simulink model "gm_PN_generator_Tx_mq"  (R2020a)
settings: Solver=FixedStepDiscrete  StartTime=0.0  StopTime=10  RelTol=1e-3
undefined symbols (not defined in the file): filt, Fs, ip, usb
libraries: commseqgen3 x2, dspmlti4 x2, plutoradiolib x1, commdigbbndpm3 x1, modelsimlib x1
settings Model: Creator=juanj  LastModifiedBy=juanj
settings OptimizationCC: BlockReduction=off  ConditionallyExecuteInputs=off  DefaultParameterBehavior=Inlined
settings DebuggingCC: AlgebraicLoopMsg=error  InheritedTsInSrcMsg=none  SingleTaskRateTransMsg=error  UnderSpecifiedDimensionMsg=warning
settings HardwareCC: ProdBitPerPointer=32  ProdBitPerSizeT=32  ProdBitPerPtrDiffT=32  ProdLargestAtomicFloat=None  ProdIntDivRoundTo=Undefined  ProdEndianess=Unspecified  ProdWordSize=32  ProdHWDeviceType=ASIC/FPGA->ASIC/FPGA  TargetBitPerPointer=64  TargetBitPerSizeT=64  TargetBitPerPtrDiffT=64  TargetLongLongMode=on  TargetIntDivRoundTo=Zero  TargetEndianess=LittleEndian  TargetWordSize=64  TargetHWDeviceType=Custom Processor->MATLAB Host Computer  ProdEqTarget=off

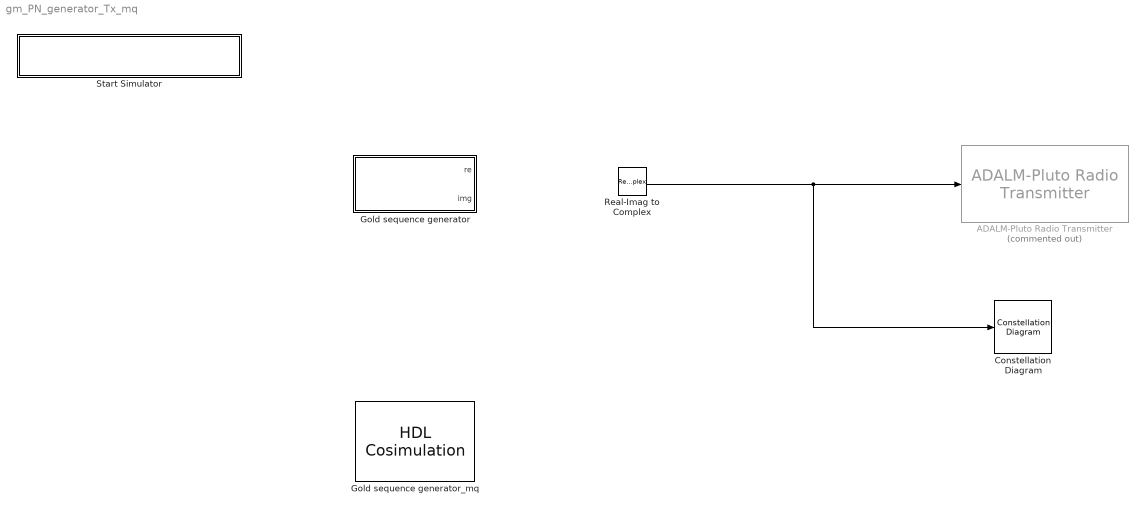
== system gm_PN_generator_Tx_mq ==
  ADALM-Pluto Radio Transmitter : plutoradiolib/ADALM-Pluto Radio Transmitter  Commented=on  RadioID=usb:0  uri=ip:10.0.0.200  CenterFrequencySource=Dialog  CenterFrequency=2.4e9  GainSource=Dialog  Gain=-10  ChannelMapping=1  BasebandSampleRate=1e6  UnderflowOutputPort=off  ShowAdvancedProperties=off  UseCustomFilter=off  filtPathRates=[737280000 11520000 3840000 1920000 960000 240000]  filtCoefficients=[-192 82 85 -215 228 -102 -110 290 -318 145 160 -426 471 -215 -238 633 -697 318 349 -923 1009 -457 -498 1309 -1423 640 693 -1812 1959 -876 -945 2458 -2647 1180 1268 -3290 3534 -1572 -1688 4375 -4698 2091 2247 -5836 6284 -2807 -3031 7918 -8588 3870 4225 -11182 12324 -5662 -6330 17255 -19735 9507 11312 -33568 43355 -25227 -42139 305542 305542 -42139 -25227 43355 -33568 11312 9507 -19735 17255 -6330 -5662 12324 -11182 4225 3870 -8588 7918 -3031 -2807 6284 -5836 2247 2091 -4698 4375 -1688 -1572 3534 -3290 1268 1180 -2647 2458 -945 -876 1959 -1812 693 640 -1423 1309 -498 -457 1009 -923 349 318 -697 633 -238 -215 471 -426 160 145 -318 290 -110 -102 228 -215 85 82 -192]  filtCoefficientSize=128  filtDecimInterpFactor=4  filtGain=-12  filtRFBandwidth=18000000  filterConfigStruct=struct()  DataSourceSelect=Input Port  DDSTone1Freq=5e3  DDSTone2Freq=10e3  DDSTone1Scale=0.5  DDSTone2Scale=0.25  DataTimeout=Inf  FrequencyCorrection=0  ENSMPinControlMode=None  BISTLoopbackMode=Disabled  BISTToneInject=Disabled  BISTSignalGen=PRBS  BISTToneFreq=Fs/32  BISTToneLevel=0
      settings: SourceProductBaseCode=PLUTO
  Constellation Diagram : ConstellationDiagram
  Gold sequence generator : Subsystem  TreatAsAtomicUnit=on
  Gold sequence generator_mq : modelsimlib/HDL Cosimulation  PortModes=[]  PortTimes=[]  PortSigns=[]  PortFracLengths=[]  CommLocal=on  CommSharedMemory=on  CommPortNumber=4449  CommShowInfo=on  ClockModes=[]  ClockTimes=[]  TclPreSimCommand=|  TclPostSimCommand="puts \"done\""  TimingMode=ns  TimingScaleFactor=10  idxCellArray={'UNUSED_VAR'}  CosimBypass=Full Simulation  AllowDirectFeedthrough=on  ProductName=EDA Simulator Link MQ  RunAutoTimescale=off  HdlClocks=0  PreRunTime=0  PreRunTimeUnit=ns
      | puts "Running Simulink Cosimulation block.";
      |  puts "Chip Name: --> PN_generator_Tx/Gold sequence generator";
      |  puts "Target language: --> vhdl";
      |  puts "Target directory: --> hdl_prj\hdlsrc\PN_generator_Tx";
      |  puts [clock format [clock seconds]];
      settings: SourceProductBaseCode=ES
  Real-Imag to Complex : RealImagToComplex
  Start Simulator : Subsystem
      settings: OpenFcn=|
      | try
      |    cosimDirName = pwd;
      |    cd 'hdl_prj\hdlsrc\PN_generator_Tx';
      |    vsim('tclstart',GoldSeque_ip_src_gm_PN_generator_Tx_mq_tcl);
      |    cd (cosimDirName);
      |    clear cosimDirName;
      | catch me
      |    disp('Failed to launch cosimulator with "vsim"');
      |    disp (me.message);
      |    cd (cosimDirName);
      |    clear cosimDirName;
      | end
      mask Display: disp(['vsimulink  -voptargs=+acc work.GoldSeque_ip' char(10) 'Double-click here to launch ModelSim'])
  wires:
  Real-Imag to Complex/1 -> Constellation Diagram/1, ADALM-Pluto Radio Transmitter/1

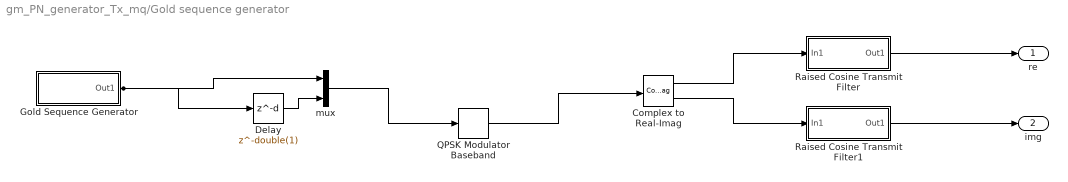
== system gm_PN_generator_Tx_mq/Gold sequence generator ==
  Complex to Real-Imag : ComplexToRealImag  SampleTime=2e-05
  Delay : Delay  DelayLength=double(1)  InitialCondition=0  SampleTime=2e-05
  Gold Sequence Generator : Subsystem  mask(Gold Sequence Generator){genPoly1='z^6 + z + 1', iniState1=[0 1 0 1 0 1], genPoly2='z^6 + z^5 + z^2 + z + 1', iniState2=[0 0 0 0 0 1], index=double(0), shift=double(0), outVarSiz=off, maxOutSizeMode=Dialog parameter, maxOutSize=[10 1], Ts=1/50000, sampPerFrame=1, reset=off, outDataType=boolean}
      mask prompts: genPoly1 "Preferred polynomial (1):"; iniState1 "Initial states (1):"; genPoly2 "Preferred polynomial (2):"; iniState2 "Initial states (2):"; index "Sequence index:"; outVarSiz "Output variable-size signals"; maxOutSizeMode "Maximum output size source:"; maxOutSize "Maximum output size:"; Ts "Sample time:"; sampPerFrame "Samples per frame:"; reset "Reset on nonzero input"; outDataType "Output data type:"
      mask help:
      | Generate a Gold sequence from a set of sequences by specifying a preferred pair of polynomials.
      |
      | The polynomial parameter values represent the shift register connections. Enter these values as either a polynomial string, a binary vector or a descending ordered polynomial to indicate the connection points.
      |
      | The sequence index parameter denotes the single sequence outputted from the set of Gold sequences. Specify it as a scalar integer in the range [-2, 2^n-2] where n is the degree of the generator polynomial. The index values -2 and -1 correspond to the first and second PN sequences as generated by the preferred polynomials (1) and (2), respectively.
      |
      | For variable-size output signals, the current output size is either specified from the 'oSiz' input or inherited from the 'Ref' input.
      mask init:
      | [eStr, genPoly1, iniState1, genPoly2, iniState2, index, shift] = commblkgcgen3(gcb, 'init', genPoly1, iniState1, genPoly2, iniState2, shift, index, sampPerFrame);
      | if (eStr.ecode == 1)
      | 	error(eStr.eID, eStr.emsg);
      | end
      | % Initial states are from the dialog always
      | iniStaSource = 1;
      mask Help: eval('blocksethelp');
      mask Callback outVarSiz: commblkgcgen3(gcb, 'cbvarsize');
      mask TypeOptions maxOutSizeMode: Dialog parameter | Inherit from reference input
      mask Callback maxOutSizeMode: commblkgcgen3(gcb,'cbmaxoutsrc');
      mask TypeOptions outDataType: double | boolean | Smallest unsigned integer
      mask Callback outDataType: commblkgcgen3(gcb,'cbOutDType');
      mask Display:
      | disp('Gold Sequence\nGenerator');
      | 
      | % Port Labels (alongwith location in normalized units)
      | vSizPortLbl.str = ''; vSizPortLbl.x = 0.0; vSizPortLbl.y = 0.0;
      | rstPortLbl.str = ''; rstPortLbl.x = 0.0; rstPortLbl.y = 0.0;
      | 
      | % Oriented positions (in normalized units) for ONLY ONE INPUT PORT
      | xRightOneInport = 0.03; yRightOneInport = 0.5;
      | xLeft_OneInport = 0.82; yLeft_OneInport = 0.5;
      | xUp___OneInport = 0.5; yUp___OneInport = 0.05;
      | xDown_OneInport = 0.5; yDown_OneInport = 0.93;
      | 
      | % Oriented positions (in normalized units) for TWO INPUT PORTS
      | xRightInport1 = 0.03; yRightInport1 = 0.75;
      | xRightInport2 = 0.03; yRightInport2 = 0.25;
      | xLeft_Inport1 = 0.82; yLeft_Inport1 = 0.75;
      | xLeft_Inport2 = 0.82; yLeft_Inport2 = 0.25;
      | xUp___Inport1 = 0.25; yUp___Inport1 = 0.05;
      | xUp___Inport2 = 0.75; yUp___Inport2 = 0.05;
      | xDown_Inport1 = 0.25; yDown_Inport1 = 0.93;
      | xDown_Inport2 = 0.75; yDown_Inport2 = 0.93;
      | 
      | blkOrientationStr = lower(get_param(gcbh, 'orientation'));
      | 
      | if (outVarSiz==0)
      |     if (reset==1) % only reset
      |         rstPortLbl.str = 'Rst';
      |         switch blkOrientationStr
      |             case 'right'
      |                 rstPortLbl.x = xRightOneInport;
      |                 rstPortLbl.y = yRightOneInport;
      |             case 'left'
      |                 rstPortLbl.x = xLeft_OneInport;
      |                 rstPortLbl.y = yLeft_OneInport;
      |             case 'up'
      |                 rstPortLbl.x = xUp___OneInport;
      |                 rstPortLbl.y = yUp___OneInport;
      |             otherwise % down
      |                 rstPortLbl.x = xDown_OneInport;
      |                 rstPortLbl.y = yDown_OneInport;
      |         end
      |     end
      | else % vSiz port on
      |     if (maxOutSizeMode==1)
      |        vSizPortLbl.str = 'oSiz';
      |     else
      |         vSizPortLbl.str = 'Ref';
      |     end
      |     if (reset==1) % both
      |         rstPortLbl.str = 'Rst';
      |         switch blkOrientationStr
      |             case 'right'
      |                 vSizPortLbl.x = xRightInport1;
      |                 vSizPortLbl.y = yRightInport1;
      |                 rstPortLbl.x = xRightInport2;
      |                 rstPortLbl.y = yRightInport2;
      |             case 'left'
      |                 vSizPortLbl.x = xLeft_Inport1;
      |                 vSizPortLbl.y = yLeft_Inport1;
      |                 rstPortLbl.x = xLeft_Inport2;
      |                 rstPortLbl.y = yLeft_Inport2;
      |             case 'up'
      |                 vSizPortLbl.x = xUp___Inport1;
      |                 vSizPortLbl.y = yUp___Inport1;
      |                 rstPortLbl.x = xUp___Inport2;
      |                 rstPortLbl.y = yUp___Inport2;
      |             otherwise % down
      |                 vSizPortLbl.x = xDown_Inport1;
      |                 vSizPortLbl.y = yDown_Inport1;
      |                 rstPortLbl.x = xDown_Inport2;
      |                 rstPortLbl.y = yDown_Inport2;
      |         end
      |     else % no reset, vSiz only
      |         switch blkOrientationStr
      |             case 'right'
      |                 vSizPortLbl.x = xRightOneInport;
      |                 vSizPortLbl.y = yRightOneInport;
      |             case 'left'
      |                 vSizPortLbl.x = xLeft_OneInport;
      |                 vSizPortLbl.y = yLeft_OneInport;
      |             case 'up'
      |                 vSizPortLbl.x = xUp___OneInport;
      |                 vSizPortLbl.y = yUp___OneInport;
      |             otherwise
      |                 vSizPortLbl.x = xDown_OneInport;
      |                 vSizPortLbl.y = yDown_OneInport;
      |         end
      |     end
      | end
      | 
      | text(vSizPortLbl.x, vSizPortLbl.y, vSizPortLbl.str);
      | text(rstPortLbl.x, rstPortLbl.y, rstPortLbl.str);
  QPSK Modulator Baseband : commdigbbndpm3/QPSK Modulator Baseband  InType=Bit  Enc=Gray  Ph=pi/4  outDtype=Fixed-point  outWordLen=16  outUDDataType=sfix(16)  outFracLenMode=Best precision  outFracLen=15  outDataTypeStr=fixdt(1,16)  outLastDataTypeStr=fixdt(1,16)
  Raised Cosine Transmit Filter : Subsystem  mask(Raised Cosine Transmit Filter){filtType=Square root, R=double(0.7), filtSpan=double(12), N=double(2), filterGain=double(1), InputProcessing=Elements as channels (sample based), RateOptions=Allow multirate processing, framing=Mute, checkCoeff=off, variableName=rcTxFilt, checkGain=Normalized, sampMode=Mute, saveAsFlag=double(0), currentFiltSpan=double(12), D=double(6), launchFVT=on, roundingMode=Floor, overflowMode=off, coeffMode=Same word length as input, coeffWordLength=double(16), coeffFracLength=double(15), coeffDataTypeStr=Inherit: Same word length as input, coeffMin=[], coeffMax=[], coeffLastDataTypeStr=Inherit: Same word length as input, prodOutputMode=Inherit via internal rule, prodOutputWordLength=double(32), prodOutputFracLength=double(30), prodOutputDataTypeStr=Inherit: Inherit via internal rule, prodOutputLastDataTypeStr=Inherit: Inherit via internal rule, accumMode=Inherit via internal rule, accumWordLength=double(32), accumFracLength=double(30), accumDataTypeStr=Inherit: Inherit via internal rule, accumLastDataTypeStr=Inherit: Inherit via internal rule, outputMode=Same as input, outputWordLength=double(16), outputFracLength=double(15), outputDataTypeStr=Inherit: Same as input, outputMin=[], outputMax=[], outputLastDataTypeStr=Inherit: Same as input, LockScale=off}
      mask prompts: filtType "Filter shape:"; R "Rolloff factor:"; filtSpan "Filter span in symbols:"; N "Output samples per symbol:"; filterGain "Linear amplitude filter gain:"; InputProcessing "dsp:FIRMultirateBlockDialog:InputProc_MP"; RateOptions "dsp:FIRMultirateBlockDialog:RateOptions_MP"; checkCoeff "Export filter coefficients to workspace"; variableName "Coefficient variable name:"; checkGain "Filter gain:"; sampMode "Input sampling mode:"; saveAsFlag "Save_as flag:"; currentFiltSpan "Current filter span in symbols:"; D "Group delay (number of symbols):"; launchFVT "Visualize filter with FVTool"; roundingMode "dspshared:FixptDialog:roundingMode"; overflowMode "Simulink:masks:SaturateOnIntegerOverflow_MP"; LockScale "dspshared:FixptDialog:lockAgnstChanges"
      mask help: Upsample and filter the input signal using a normal or square root raised cosine FIR filter.
      mask init:
      | commblkrcfilttx(gcbh,'frameupgrademultirate');
      | 
      | [filt, icon, err] = commblkrcfilttx(gcbh,'init',...
      |     filtType, R, filtSpan, currentFiltSpan, D, N, filterGain, ...
      |     checkCoeff, variableName);
      | 
      | % Set sample modes of underlying blocks
      | commblkrcfilttx(gcb,'setFIRInterp', InputProcessing, RateOptions, ...
      |     roundingMode, overflowMode, LockScale);
      | 
      | if(~isempty(err.msg))
      | 	error(err.eID,err.msg);
      | end
      mask Help: eval('blocksethelp');
      mask TypeOptions filtType: Normal | Square root
      mask TypeOptions InputProcessing: Columns as channels (frame based) | Elements as channels (sample based)
      mask Callback InputProcessing: commblkrcfilttx(gcbh,'cbInputProcessing');
      mask TypeOptions RateOptions: Enforce single-rate processing | Allow multirate processing
      mask TypeOptions framing: Enforce single-rate processing | Allow multirate processing | Maintain input frame rate | Maintain input frame size | Mute
      mask Callback checkCoeff: commblkrcfilttx(gcbh,'cbCheckCoeff');
      mask Callback variableName: commblkrcfilttx(gcbh,'dialogdynamic');
      mask TypeOptions checkGain: Normalized | User-specified
      mask TypeOptions sampMode: Frame-based | Sample-based | Mute
      mask TypeOptions roundingMode: Ceiling | Convergent | Floor | Nearest | Round | Simplest | Zero
      mask TypeOptions coeffMode: Same word length as input | Specify word length | Binary point scaling | Slope and bias scaling
      mask TypeOptions prodOutputMode: Inherit via internal rule | Same as input | Binary point scaling | Slope and bias scaling
      mask TypeOptions accumMode: Inherit via internal rule | Same as product output | Same as input | Binary point scaling | Slope and bias scaling
      mask TypeOptions outputMode: Same as accumulator | Same as product output | Same as input | Binary point scaling | Slope and bias scaling
      mask Display:
      | plot(0,0,1,1,icon.xx,icon.plot);
      | text(icon.x,icon.y,icon.str,'horiz','center');
  Raised Cosine Transmit Filter1 : Subsystem  mask(Raised Cosine Transmit Filter){filtType=Square root, R=double(0.7), filtSpan=double(12), N=double(2), filterGain=double(1), InputProcessing=Elements as channels (sample based), RateOptions=Allow multirate processing, framing=Mute, checkCoeff=off, variableName=rcTxFilt1, checkGain=Normalized, sampMode=Mute, saveAsFlag=double(0), currentFiltSpan=double(12), D=double(6), launchFVT=on, roundingMode=Floor, overflowMode=off, coeffMode=Same word length as input, coeffWordLength=double(16), coeffFracLength=double(15), coeffDataTypeStr=Inherit: Same word length as input, coeffMin=[], coeffMax=[], coeffLastDataTypeStr=Inherit: Same word length as input, prodOutputMode=Inherit via internal rule, prodOutputWordLength=double(32), prodOutputFracLength=double(30), prodOutputDataTypeStr=Inherit: Inherit via internal rule, prodOutputLastDataTypeStr=Inherit: Inherit via internal rule, accumMode=Inherit via internal rule, accumWordLength=double(32), accumFracLength=double(30), accumDataTypeStr=Inherit: Inherit via internal rule, accumLastDataTypeStr=Inherit: Inherit via internal rule, outputMode=Same as input, outputWordLength=double(16), outputFracLength=double(15), outputDataTypeStr=Inherit: Same as input, outputMin=[], outputMax=[], outputLastDataTypeStr=Inherit: Same as input, LockScale=off}
      mask prompts: filtType "Filter shape:"; R "Rolloff factor:"; filtSpan "Filter span in symbols:"; N "Output samples per symbol:"; filterGain "Linear amplitude filter gain:"; InputProcessing "dsp:FIRMultirateBlockDialog:InputProc_MP"; RateOptions "dsp:FIRMultirateBlockDialog:RateOptions_MP"; checkCoeff "Export filter coefficients to workspace"; variableName "Coefficient variable name:"; checkGain "Filter gain:"; sampMode "Input sampling mode:"; saveAsFlag "Save_as flag:"; currentFiltSpan "Current filter span in symbols:"; D "Group delay (number of symbols):"; launchFVT "Visualize filter with FVTool"; roundingMode "dspshared:FixptDialog:roundingMode"; overflowMode "Simulink:masks:SaturateOnIntegerOverflow_MP"; LockScale "dspshared:FixptDialog:lockAgnstChanges"
      mask help: Upsample and filter the input signal using a normal or square root raised cosine FIR filter.
      mask init: same as gm_PN_generator_Tx_mq/Gold sequence generator/Raised Cosine Transmit Filter
      mask Help: eval('blocksethelp');
      mask TypeOptions filtType: Normal | Square root
      mask TypeOptions InputProcessing: Columns as channels (frame based) | Elements as channels (sample based)
      mask Callback InputProcessing: commblkrcfilttx(gcbh,'cbInputProcessing');
      mask TypeOptions RateOptions: Enforce single-rate processing | Allow multirate processing
      mask TypeOptions framing: Enforce single-rate processing | Allow multirate processing | Maintain input frame rate | Maintain input frame size | Mute
      mask Callback checkCoeff: commblkrcfilttx(gcbh,'cbCheckCoeff');
      mask Callback variableName: commblkrcfilttx(gcbh,'dialogdynamic');
      mask TypeOptions checkGain: Normalized | User-specified
      mask TypeOptions sampMode: Frame-based | Sample-based | Mute
      mask TypeOptions roundingMode: Ceiling | Convergent | Floor | Nearest | Round | Simplest | Zero
      mask TypeOptions coeffMode: Same word length as input | Specify word length | Binary point scaling | Slope and bias scaling
      mask TypeOptions prodOutputMode: Inherit via internal rule | Same as input | Binary point scaling | Slope and bias scaling
      mask TypeOptions accumMode: Inherit via internal rule | Same as product output | Same as input | Binary point scaling | Slope and bias scaling
      mask TypeOptions outputMode: Same as accumulator | Same as product output | Same as input | Binary point scaling | Slope and bias scaling
      mask Display:
      | plot(0,0,1,1,icon.xx,icon.plot);
      | text(icon.x,icon.y,icon.str,'horiz','center');
  mux : Mux  Inputs=2
  re : Outport
  img : Outport  Port=2  VectorParamsAs1DForOutWhenUnconnected=off
  wires:
  mux/1 -> QPSK Modulator Baseband/1
  Complex to Real-Imag/2 -> Raised Cosine Transmit Filter1/1(In1)
  Complex to Real-Imag/1 -> Raised Cosine Transmit Filter/1(In1)
  Raised Cosine Transmit Filter1/1(Out1) -> img/1
  Raised Cosine Transmit Filter/1(Out1) -> re/1
  QPSK Modulator Baseband/1 -> Complex to Real-Imag/1
  Gold Sequence Generator/1(Out1) -> mux/1, Delay/1
  Delay/1 -> mux/2

== system gm_PN_generator_Tx_mq/Start Simulator ==

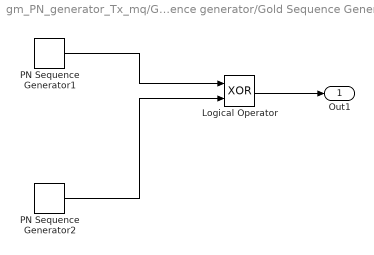
== system gm_PN_generator_Tx_mq/Gold sequence generator/Gold Sequence Generator ==
  Logical Operator : Logic  Operator=XOR  AllPortsSameDT=off  OutDataTypeStr=boolean  SampleTime=2e-05
  PN Sequence Generator1 : commseqgen3/PN Sequence Generator  poly=genPoly1  ini_sta=iniState1  outBitMaskSource=Dialog parameter  shift=shift  outVarSiz=off  maxOutSizeMode=Dialog parameter  maxOutSize=maxOutSize  Ts=Ts  sampPerFrame=sampPerFrame  reset=off  bitPackedOutputs=off  outDataType=boolean  numPackedBits=8  bitPackDataSigned=off  bitPackedOutDType=double
  PN Sequence Generator2 : commseqgen3/PN Sequence Generator  poly=genPoly2  ini_sta=iniState2  outBitMaskSource=Dialog parameter  shift=shift + index  outVarSiz=off  maxOutSizeMode=Dialog parameter  maxOutSize=maxOutSize  Ts=Ts  sampPerFrame=sampPerFrame  reset=off  bitPackedOutputs=off  outDataType=boolean  numPackedBits=8  bitPackDataSigned=off  bitPackedOutDType=double
  Out1 : Outport
  wires:
  PN Sequence Generator2/1 -> Logical Operator/2
  PN Sequence Generator1/1 -> Logical Operator/1
  Logical Operator/1 -> Out1/1

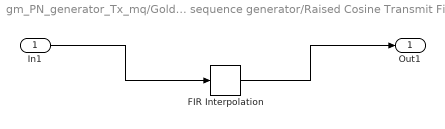
== system gm_PN_generator_Tx_mq/Gold sequence generator/Raised Cosine Transmit Filter ==
  In1 : Inport  OutDataTypeStr=fixdt(1, 16, 15)  SampleTime=2e-05
  FIR Interpolation : dspmlti4/FIR Interpolation  FilterSource=Dialog parameters  PrivateCoeffs=0  h=filt.coeff  L=filt.rateFactor  FilterObject=Hm_firinterp  framing=Allow multirate processing  outputBufInitCond=0  roundingMode=Floor  overflowMode=off  firstCoeffDataTypeStr=Inherit: Same word length as input  firstCoeffMin=[]  firstCoeffMax=[]  firstCoeffLastDataTypeStr=Inherit: Same word length as input  outputMin=[]  outputMax=[]
  Out1 : Outport
  wires:
  In1/1 -> FIR Interpolation/1
  FIR Interpolation/1 -> Out1/1

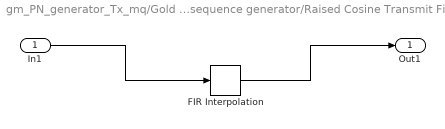
== system gm_PN_generator_Tx_mq/Gold sequence generator/Raised Cosine Transmit Filter1 ==
  In1 : Inport  OutDataTypeStr=fixdt(1, 16, 15)  SampleTime=2e-05
  FIR Interpolation : dspmlti4/FIR Interpolation  FilterSource=Dialog parameters  PrivateCoeffs=0  h=filt.coeff  L=filt.rateFactor  FilterObject=Hm_firinterp  framing=Allow multirate processing  outputBufInitCond=0  roundingMode=Floor  overflowMode=off  firstCoeffDataTypeStr=Inherit: Same word length as input  firstCoeffMin=[]  firstCoeffMax=[]  firstCoeffLastDataTypeStr=Inherit: Same word length as input  outputMin=[]  outputMax=[]
  Out1 : Outport
  wires:
  In1/1 -> FIR Interpolation/1
  FIR Interpolation/1 -> Out1/1
